simulink model "Main_Project"  (R2016a)
settings: Solver=ode4  StartTime=0.0  StopTime=100  FixedStep=0.001  MaxStep=0.01  RelTol=1e-6
values from neighbouring files (symbols this model uses):
  float =     [waveglider.mat]
  floatABC =     [waveglider.mat]
  gliderABC =     [waveglider.mat]
undefined symbols (not defined in the file or in its folder): magnitude, RAO_Vel
libraries: simulink_extras x8, marine_gnc x4, simulink x4, marine_hydro x1
(part 3 of 3)

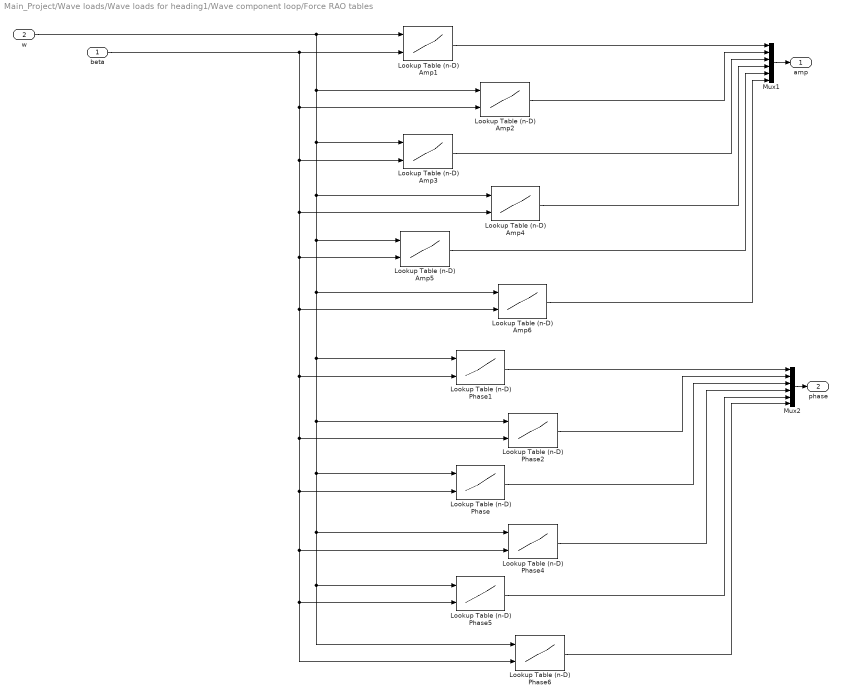
== system Main_Project/Wave loads/Wave loads for heading1/Wave component loop/Force RAO tables ==
  beta : Inport
  w : Inport  Port=2
  Lookup Table (n-D) Amp1 : Lookup_n-D  BreakpointsForDimension1=float.forceRAO.w  BreakpointsForDimension2=float.headings  BreakpointsForDimension3=RAO_Vel  IndexSearchMethod=Linear search  BeginIndexSearchUsingPreviousIndexResult=on  Table=float.forceRAO.amp{1}  ExtrapMethod=Clip  DiagnosticForOutOfRangeInput=Warning  InternalRulePriority=Speed  RndMeth=Simplest  InputSameDT=on
  Lookup Table (n-D) Amp2 : Lookup_n-D  BreakpointsForDimension1=float.forceRAO.w  BreakpointsForDimension2=float.headings  BreakpointsForDimension3=RAO_Vel  IndexSearchMethod=Linear search  BeginIndexSearchUsingPreviousIndexResult=on  Table=float.forceRAO.amp{2}  ExtrapMethod=Clip  DiagnosticForOutOfRangeInput=Warning  InternalRulePriority=Speed  RndMeth=Simplest  InputSameDT=on
  Lookup Table (n-D) Amp3 : Lookup_n-D  BreakpointsForDimension1=float.forceRAO.w  BreakpointsForDimension2=float.headings  BreakpointsForDimension3=RAO_Vel  IndexSearchMethod=Linear search  BeginIndexSearchUsingPreviousIndexResult=on  Table=float.forceRAO.amp{3}  ExtrapMethod=Clip  DiagnosticForOutOfRangeInput=Warning  InternalRulePriority=Speed  RndMeth=Simplest  InputSameDT=on
  Lookup Table (n-D) Amp4 : Lookup_n-D  BreakpointsForDimension1=float.forceRAO.w  BreakpointsForDimension2=float.headings  BreakpointsForDimension3=RAO_Vel  IndexSearchMethod=Linear search  BeginIndexSearchUsingPreviousIndexResult=on  Table=float.forceRAO.amp{4}  ExtrapMethod=Clip  DiagnosticForOutOfRangeInput=Warning  InternalRulePriority=Speed  RndMeth=Simplest  InputSameDT=on
  Lookup Table (n-D) Amp5 : Lookup_n-D  BreakpointsForDimension1=float.forceRAO.w  BreakpointsForDimension2=float.headings  BreakpointsForDimension3=RAO_Vel  IndexSearchMethod=Linear search  BeginIndexSearchUsingPreviousIndexResult=on  Table=float.forceRAO.amp{5}  ExtrapMethod=Clip  DiagnosticForOutOfRangeInput=Warning  InternalRulePriority=Speed  RndMeth=Simplest  InputSameDT=on
  Lookup Table (n-D) Amp6 : Lookup_n-D  BreakpointsForDimension1=float.forceRAO.w  BreakpointsForDimension2=float.headings  BreakpointsForDimension3=RAO_Vel  IndexSearchMethod=Linear search  BeginIndexSearchUsingPreviousIndexResult=on  Table=float.forceRAO.amp{6}  ExtrapMethod=Clip  DiagnosticForOutOfRangeInput=Warning  InternalRulePriority=Speed  RndMeth=Simplest  InputSameDT=on
  Lookup Table (n-D) Phase : Lookup_n-D  BreakpointsForDimension1=float.forceRAO.w  BreakpointsForDimension2=float.headings  BreakpointsForDimension3=RAO_Vel  IndexSearchMethod=Linear search  BeginIndexSearchUsingPreviousIndexResult=on  Table=float.forceRAO.phase{3}  ExtrapMethod=Clip  DiagnosticForOutOfRangeInput=Warning  InternalRulePriority=Speed  RndMeth=Simplest  InputSameDT=on
  Lookup Table (n-D) Phase1 : Lookup_n-D  BreakpointsForDimension1=float.forceRAO.w  BreakpointsForDimension2=float.headings  BreakpointsForDimension3=RAO_Vel  IndexSearchMethod=Linear search  BeginIndexSearchUsingPreviousIndexResult=on  Table=float.forceRAO.phase{1}  ExtrapMethod=Clip  DiagnosticForOutOfRangeInput=Warning  InternalRulePriority=Speed  RndMeth=Simplest  InputSameDT=on
  Lookup Table (n-D) Phase2 : Lookup_n-D  BreakpointsForDimension1=float.forceRAO.w  BreakpointsForDimension2=float.headings  BreakpointsForDimension3=RAO_Vel  IndexSearchMethod=Linear search  BeginIndexSearchUsingPreviousIndexResult=on  Table=float.forceRAO.phase{2}  ExtrapMethod=Clip  DiagnosticForOutOfRangeInput=Warning  InternalRulePriority=Speed  RndMeth=Simplest  InputSameDT=on
  Lookup Table (n-D) Phase4 : Lookup_n-D  BreakpointsForDimension1=float.forceRAO.w  BreakpointsForDimension2=float.headings  BreakpointsForDimension3=RAO_Vel  IndexSearchMethod=Linear search  BeginIndexSearchUsingPreviousIndexResult=on  Table=float.forceRAO.phase{4}  ExtrapMethod=Clip  DiagnosticForOutOfRangeInput=Warning  InternalRulePriority=Speed  RndMeth=Simplest  InputSameDT=on
  Lookup Table (n-D) Phase5 : Lookup_n-D  BreakpointsForDimension1=float.forceRAO.w  BreakpointsForDimension2=float.headings  BreakpointsForDimension3=RAO_Vel  IndexSearchMethod=Linear search  BeginIndexSearchUsingPreviousIndexResult=on  Table=float.forceRAO.phase{5}  ExtrapMethod=Clip  DiagnosticForOutOfRangeInput=Warning  InternalRulePriority=Speed  RndMeth=Simplest  InputSameDT=on
  Lookup Table (n-D) Phase6 : Lookup_n-D  BreakpointsForDimension1=float.forceRAO.w  BreakpointsForDimension2=float.headings  BreakpointsForDimension3=RAO_Vel  IndexSearchMethod=Linear search  BeginIndexSearchUsingPreviousIndexResult=on  Table=float.forceRAO.phase{6}  ExtrapMethod=Clip  DiagnosticForOutOfRangeInput=Warning  InternalRulePriority=Speed  RndMeth=Simplest  InputSameDT=on
  Mux1 : Mux  Inputs=6
  Mux2 : Mux  Inputs=6
  amp : Outport
  phase : Outport  Port=2
  wires:
  w/1 -> Lookup Table (n-D) Amp1/1, Lookup Table (n-D) Amp2/1, Lookup Table (n-D) Amp3/1, Lookup Table (n-D) Amp4/1, Lookup Table (n-D) Amp5/1, Lookup Table (n-D) Amp6/1, Lookup Table (n-D) Phase1/1, Lookup Table (n-D) Phase2/1, Lookup Table (n-D) Phase/1, Lookup Table (n-D) Phase4/1, Lookup Table (n-D) Phase6/1, Lookup Table (n-D) Phase5/1
  Lookup Table (n-D) Phase5/1 -> Mux2/5
  Lookup Table (n-D) Phase/1 -> Mux2/3
  Lookup Table (n-D) Phase1/1 -> Mux2/1
  beta/1 -> Lookup Table (n-D) Amp1/2, Lookup Table (n-D) Amp2/2, Lookup Table (n-D) Amp3/2, Lookup Table (n-D) Amp4/2, Lookup Table (n-D) Amp6/2, Lookup Table (n-D) Phase1/2, Lookup Table (n-D) Phase2/2, Lookup Table (n-D) Phase/2, Lookup Table (n-D) Phase4/2, Lookup Table (n-D) Phase6/2, Lookup Table (n-D) Phase5/2, Lookup Table (n-D) Amp5/2
  Lookup Table (n-D) Phase4/1 -> Mux2/4
  Lookup Table (n-D) Phase2/1 -> Mux2/2
  Lookup Table (n-D) Phase6/1 -> Mux2/6
  Lookup Table (n-D) Amp4/1 -> Mux1/4
  Lookup Table (n-D) Amp1/1 -> Mux1/1
  Lookup Table (n-D) Amp3/1 -> Mux1/3
  Lookup Table (n-D) Amp5/1 -> Mux1/5
  Lookup Table (n-D) Amp2/1 -> Mux1/2
  Lookup Table (n-D) Amp6/1 -> Mux1/6
  Mux2/1 -> phase/1
  Mux1/1 -> amp/1

== system Main_Project/Wave loads/Wave loads for heading1/Wave component loop/WD RAO tables ==
  beta : Inport
  w : Inport  Port=2
  Constant : Constant  Value=0
  Lookup Table (n-D) Wavedrift 1 : Lookup_n-D  BreakpointsForDimension1=float.driftfrc.w  BreakpointsForDimension2=float.headings  BreakpointsForDimension3=RAO_Vel  IndexSearchMethod=Linear search  BeginIndexSearchUsingPreviousIndexResult=on  Table=float.driftfrc.amp{1}  ExtrapMethod=Clip  DiagnosticForOutOfRangeInput=Warning  InternalRulePriority=Speed  RndMeth=Simplest  InputSameDT=on
  Lookup Table (n-D) Wavedrift 2 : Lookup_n-D  BreakpointsForDimension1=float.driftfrc.w  BreakpointsForDimension2=float.headings  BreakpointsForDimension3=RAO_Vel  IndexSearchMethod=Linear search  BeginIndexSearchUsingPreviousIndexResult=on  Table=float.driftfrc.amp{2}  ExtrapMethod=Clip  DiagnosticForOutOfRangeInput=Warning  InternalRulePriority=Speed  RndMeth=Simplest  InputSameDT=on
  Lookup Table (n-D) Wavedrift 3 : Lookup_n-D  BreakpointsForDimension1=float.driftfrc.w  BreakpointsForDimension2=float.headings  BreakpointsForDimension3=RAO_Vel  IndexSearchMethod=Linear search  BeginIndexSearchUsingPreviousIndexResult=on  Table=float.driftfrc.amp{3}  ExtrapMethod=Clip  DiagnosticForOutOfRangeInput=Warning  InternalRulePriority=Speed  RndMeth=Simplest  InputSameDT=on
  Mux1 : Mux  Inputs=6
  amp : Outport
  wires:
  w/1 -> Lookup Table (n-D) Wavedrift 1/1, Lookup Table (n-D) Wavedrift 3/1, Lookup Table (n-D) Wavedrift 2/1
  Constant/1 -> Mux1/5, Mux1/4, Mux1/3
  beta/1 -> Lookup Table (n-D) Wavedrift 1/2, Lookup Table (n-D) Wavedrift 3/2, Lookup Table (n-D) Wavedrift 2/2
  Lookup Table (n-D) Wavedrift 1/1 -> Mux1/1
  Lookup Table (n-D) Wavedrift 2/1 -> Mux1/2
  Lookup Table (n-D) Wavedrift 3/1 -> Mux1/6
  Mux1/1 -> amp/1

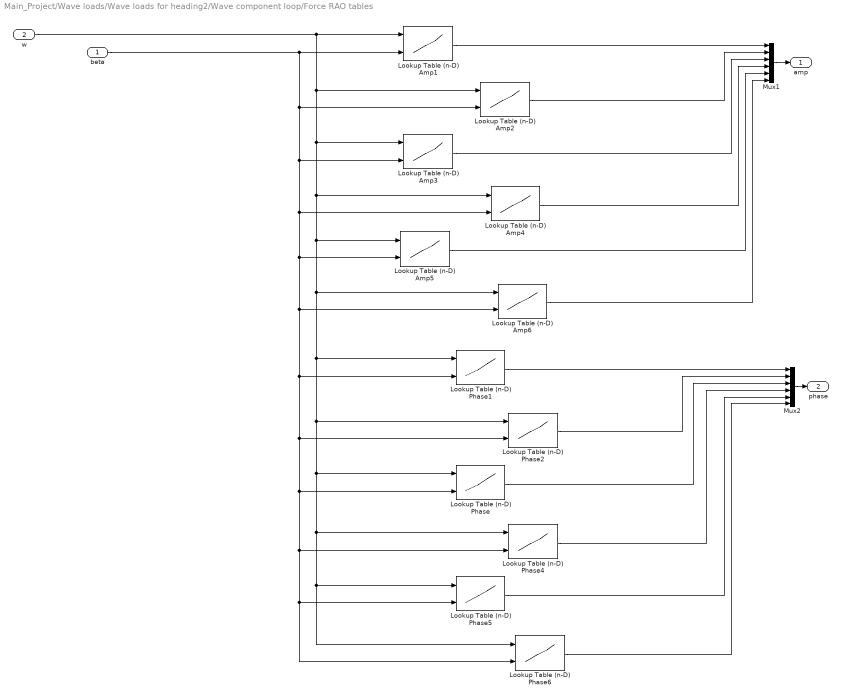
== system Main_Project/Wave loads/Wave loads for heading2/Wave component loop/Force RAO tables ==
  beta : Inport
  w : Inport  Port=2
  Lookup Table (n-D) Amp1 : Lookup_n-D  BreakpointsForDimension1=float.forceRAO.w  BreakpointsForDimension2=float.headings  BreakpointsForDimension3=RAO_Vel  IndexSearchMethod=Linear search  BeginIndexSearchUsingPreviousIndexResult=on  Table=float.forceRAO.amp{1}  ExtrapMethod=Clip  DiagnosticForOutOfRangeInput=Warning  InternalRulePriority=Speed  RndMeth=Simplest  InputSameDT=on
  Lookup Table (n-D) Amp2 : Lookup_n-D  BreakpointsForDimension1=float.forceRAO.w  BreakpointsForDimension2=float.headings  BreakpointsForDimension3=RAO_Vel  IndexSearchMethod=Linear search  BeginIndexSearchUsingPreviousIndexResult=on  Table=float.forceRAO.amp{2}  ExtrapMethod=Clip  DiagnosticForOutOfRangeInput=Warning  InternalRulePriority=Speed  RndMeth=Simplest  InputSameDT=on
  Lookup Table (n-D) Amp3 : Lookup_n-D  BreakpointsForDimension1=float.forceRAO.w  BreakpointsForDimension2=float.headings  BreakpointsForDimension3=RAO_Vel  IndexSearchMethod=Linear search  BeginIndexSearchUsingPreviousIndexResult=on  Table=float.forceRAO.amp{3}  ExtrapMethod=Clip  DiagnosticForOutOfRangeInput=Warning  InternalRulePriority=Speed  RndMeth=Simplest  InputSameDT=on
  Lookup Table (n-D) Amp4 : Lookup_n-D  BreakpointsForDimension1=float.forceRAO.w  BreakpointsForDimension2=float.headings  BreakpointsForDimension3=RAO_Vel  IndexSearchMethod=Linear search  BeginIndexSearchUsingPreviousIndexResult=on  Table=float.forceRAO.amp{4}  ExtrapMethod=Clip  DiagnosticForOutOfRangeInput=Warning  InternalRulePriority=Speed  RndMeth=Simplest  InputSameDT=on
  Lookup Table (n-D) Amp5 : Lookup_n-D  BreakpointsForDimension1=float.forceRAO.w  BreakpointsForDimension2=float.headings  BreakpointsForDimension3=RAO_Vel  IndexSearchMethod=Linear search  BeginIndexSearchUsingPreviousIndexResult=on  Table=float.forceRAO.amp{5}  ExtrapMethod=Clip  DiagnosticForOutOfRangeInput=Warning  InternalRulePriority=Speed  RndMeth=Simplest  InputSameDT=on
  Lookup Table (n-D) Amp6 : Lookup_n-D  BreakpointsForDimension1=float.forceRAO.w  BreakpointsForDimension2=float.headings  BreakpointsForDimension3=RAO_Vel  IndexSearchMethod=Linear search  BeginIndexSearchUsingPreviousIndexResult=on  Table=float.forceRAO.amp{6}  ExtrapMethod=Clip  DiagnosticForOutOfRangeInput=Warning  InternalRulePriority=Speed  RndMeth=Simplest  InputSameDT=on
  Lookup Table (n-D) Phase : Lookup_n-D  BreakpointsForDimension1=float.forceRAO.w  BreakpointsForDimension2=float.headings  BreakpointsForDimension3=RAO_Vel  IndexSearchMethod=Linear search  BeginIndexSearchUsingPreviousIndexResult=on  Table=float.forceRAO.phase{3}  ExtrapMethod=Clip  DiagnosticForOutOfRangeInput=Warning  InternalRulePriority=Speed  RndMeth=Simplest  InputSameDT=on
  Lookup Table (n-D) Phase1 : Lookup_n-D  BreakpointsForDimension1=float.forceRAO.w  BreakpointsForDimension2=float.headings  BreakpointsForDimension3=RAO_Vel  IndexSearchMethod=Linear search  BeginIndexSearchUsingPreviousIndexResult=on  Table=float.forceRAO.phase{1}  ExtrapMethod=Clip  DiagnosticForOutOfRangeInput=Warning  InternalRulePriority=Speed  RndMeth=Simplest  InputSameDT=on
  Lookup Table (n-D) Phase2 : Lookup_n-D  BreakpointsForDimension1=float.forceRAO.w  BreakpointsForDimension2=float.headings  BreakpointsForDimension3=RAO_Vel  IndexSearchMethod=Linear search  BeginIndexSearchUsingPreviousIndexResult=on  Table=float.forceRAO.phase{2}  ExtrapMethod=Clip  DiagnosticForOutOfRangeInput=Warning  InternalRulePriority=Speed  RndMeth=Simplest  InputSameDT=on
  Lookup Table (n-D) Phase4 : Lookup_n-D  BreakpointsForDimension1=float.forceRAO.w  BreakpointsForDimension2=float.headings  BreakpointsForDimension3=RAO_Vel  IndexSearchMethod=Linear search  BeginIndexSearchUsingPreviousIndexResult=on  Table=float.forceRAO.phase{4}  ExtrapMethod=Clip  DiagnosticForOutOfRangeInput=Warning  InternalRulePriority=Speed  RndMeth=Simplest  InputSameDT=on
  Lookup Table (n-D) Phase5 : Lookup_n-D  BreakpointsForDimension1=float.forceRAO.w  BreakpointsForDimension2=float.headings  BreakpointsForDimension3=RAO_Vel  IndexSearchMethod=Linear search  BeginIndexSearchUsingPreviousIndexResult=on  Table=float.forceRAO.phase{5}  ExtrapMethod=Clip  DiagnosticForOutOfRangeInput=Warning  InternalRulePriority=Speed  RndMeth=Simplest  InputSameDT=on
  Lookup Table (n-D) Phase6 : Lookup_n-D  BreakpointsForDimension1=float.forceRAO.w  BreakpointsForDimension2=float.headings  BreakpointsForDimension3=RAO_Vel  IndexSearchMethod=Linear search  BeginIndexSearchUsingPreviousIndexResult=on  Table=float.forceRAO.phase{6}  ExtrapMethod=Clip  DiagnosticForOutOfRangeInput=Warning  InternalRulePriority=Speed  RndMeth=Simplest  InputSameDT=on
  Mux1 : Mux  Inputs=6
  Mux2 : Mux  Inputs=6
  amp : Outport
  phase : Outport  Port=2
  wires:
  w/1 -> Lookup Table (n-D) Amp1/1, Lookup Table (n-D) Amp2/1, Lookup Table (n-D) Amp3/1, Lookup Table (n-D) Amp4/1, Lookup Table (n-D) Amp5/1, Lookup Table (n-D) Amp6/1, Lookup Table (n-D) Phase1/1, Lookup Table (n-D) Phase2/1, Lookup Table (n-D) Phase/1, Lookup Table (n-D) Phase4/1, Lookup Table (n-D) Phase6/1, Lookup Table (n-D) Phase5/1
  Lookup Table (n-D) Phase5/1 -> Mux2/5
  Lookup Table (n-D) Phase/1 -> Mux2/3
  Lookup Table (n-D) Phase1/1 -> Mux2/1
  beta/1 -> Lookup Table (n-D) Amp1/2, Lookup Table (n-D) Amp2/2, Lookup Table (n-D) Amp3/2, Lookup Table (n-D) Amp4/2, Lookup Table (n-D) Amp6/2, Lookup Table (n-D) Phase1/2, Lookup Table (n-D) Phase2/2, Lookup Table (n-D) Phase/2, Lookup Table (n-D) Phase4/2, Lookup Table (n-D) Phase6/2, Lookup Table (n-D) Phase5/2, Lookup Table (n-D) Amp5/2
  Lookup Table (n-D) Phase4/1 -> Mux2/4
  Lookup Table (n-D) Phase2/1 -> Mux2/2
  Lookup Table (n-D) Phase6/1 -> Mux2/6
  Lookup Table (n-D) Amp4/1 -> Mux1/4
  Lookup Table (n-D) Amp1/1 -> Mux1/1
  Lookup Table (n-D) Amp3/1 -> Mux1/3
  Lookup Table (n-D) Amp5/1 -> Mux1/5
  Lookup Table (n-D) Amp2/1 -> Mux1/2
  Lookup Table (n-D) Amp6/1 -> Mux1/6
  Mux2/1 -> phase/1
  Mux1/1 -> amp/1

== system Main_Project/Wave loads/Wave loads for heading2/Wave component loop/WD RAO tables ==
  beta : Inport
  w : Inport  Port=2
  Constant : Constant  Value=0
  Lookup Table (n-D) Wavedrift 1 : Lookup_n-D  BreakpointsForDimension1=float.driftfrc.w  BreakpointsForDimension2=float.headings  BreakpointsForDimension3=RAO_Vel  IndexSearchMethod=Linear search  BeginIndexSearchUsingPreviousIndexResult=on  Table=float.driftfrc.amp{1}  ExtrapMethod=Clip  DiagnosticForOutOfRangeInput=Warning  InternalRulePriority=Speed  RndMeth=Simplest  InputSameDT=on
  Lookup Table (n-D) Wavedrift 2 : Lookup_n-D  BreakpointsForDimension1=float.driftfrc.w  BreakpointsForDimension2=float.headings  BreakpointsForDimension3=RAO_Vel  IndexSearchMethod=Linear search  BeginIndexSearchUsingPreviousIndexResult=on  Table=float.driftfrc.amp{2}  ExtrapMethod=Clip  DiagnosticForOutOfRangeInput=Warning  InternalRulePriority=Speed  RndMeth=Simplest  InputSameDT=on
  Lookup Table (n-D) Wavedrift 3 : Lookup_n-D  BreakpointsForDimension1=float.driftfrc.w  BreakpointsForDimension2=float.headings  BreakpointsForDimension3=RAO_Vel  IndexSearchMethod=Linear search  BeginIndexSearchUsingPreviousIndexResult=on  Table=float.driftfrc.amp{3}  ExtrapMethod=Clip  DiagnosticForOutOfRangeInput=Warning  InternalRulePriority=Speed  RndMeth=Simplest  InputSameDT=on
  Mux1 : Mux  Inputs=6
  amp : Outport
  wires:
  w/1 -> Lookup Table (n-D) Wavedrift 1/1, Lookup Table (n-D) Wavedrift 3/1, Lookup Table (n-D) Wavedrift 2/1
  Constant/1 -> Mux1/5, Mux1/4, Mux1/3
  beta/1 -> Lookup Table (n-D) Wavedrift 1/2, Lookup Table (n-D) Wavedrift 3/2, Lookup Table (n-D) Wavedrift 2/2
  Lookup Table (n-D) Wavedrift 1/1 -> Mux1/1
  Lookup Table (n-D) Wavedrift 2/1 -> Mux1/2
  Lookup Table (n-D) Wavedrift 3/1 -> Mux1/6
  Mux1/1 -> amp/1

== matlab function Main_Project/Rudder/MATLAB Function ==
  data: alpha input; Cl output; Cdc input; lamda input; eks input
function Cl = fcn(alpha,Cdc,lamda,eks)
%#codegen

Cl = 1.8*pi*lamda*alpha/(cos(eks)*sqrt(lamda^2/cos(eks)^4+4)+1.8)+Cdc*alpha^2/lamda;

== matlab function Main_Project/tether tension/MATLAB Function ==
  data: x input; T output; y input; z input; alpha output; beta output
function [T,alpha,beta] = fcn(x,y,z)
%#codegen
T=1.7e+7*(sqrt(x^2+y^2+z^2)-6.2)+200;
if T<0
    T=0;
end
alpha=0;
if x>0
    alpha=atan(y/x);
elseif x<0
    alpha=atan(y/x)+pi;
elseif x==0
    if y>0
        alpha=pi/2;
    elseif y==0
        alpha=0;
    else alpha=-pi/2;
    end
end
beta=asin(sqrt((x^2+y^2)/(x^2+y^2+z^2)));

== matlab function Main_Project/Hydrofoil force/steady foilforce/MATLAB Function ==
  data: alpha input; CL output; Cdc input; lamda input; eks input
function CL = fcn(alpha,Cdc,lamda,eks)
%#codegen

CL = 1.8*pi*lamda*alpha/(cos(eks)*sqrt(lamda^2/cos(eks)^4+4)+1.8)+Cdc*alpha^2/lamda;
